simulink model "helicoptertest"  (R2022b)
settings: Solver=FixedStepAuto  StartTime=0.0  StopTime=60.0  FixedStep=0.01  RelTol=1e-3
settings Model: Creator=22438  LastModifiedBy=22438

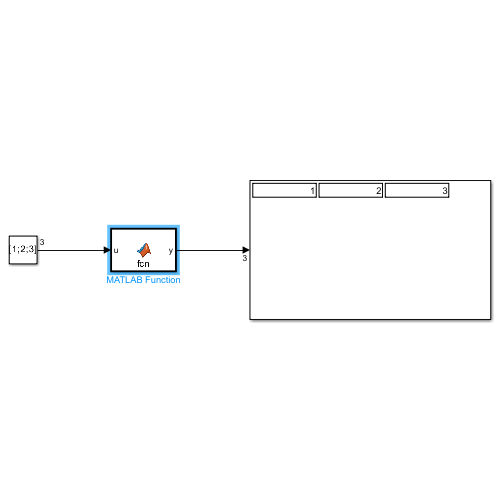
[thumbnail: Simulink's stored preview of the top-level diagram]
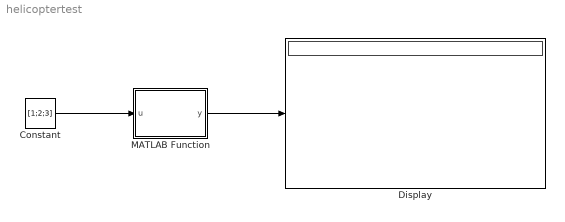
== system helicoptertest ==
  Constant : Constant  Value=[1;2;3]
  Display : Display
  MATLAB Function : MATLAB Function  TreatAsAtomicUnit=on
  wires:
  Constant/1 -> MATLAB Function/1(u)
  MATLAB Function/1(y) -> Display/1

== matlab function helicoptertest/MATLAB Function ==
  data: u input; y output
function y = fcn(u)

y = u*[1 2 3];
end
